simulink model "IntegratedStarterGenerator"  (R2024b)
settings: Solver=ode23tb  StartTime=0.0  StopTime=10  FixedStep=1e-6  RelTol=1e-4  EnableMultiTasking=on
PreLoadFcn:
  | BeltStarterGeneratorData;
model workspace (MAT data in the model file):
  Cdc = 0.001
  ID_MAP = [-155.095933536 -155.095933536 -155.095933536 -155.095933536 -155.095933536 -155.095933536 -155.095933536 -155.095933536 -200.847752045 -245.560073478 -288.511134519 -330.698372533 ... (48076 elements, 28x101x17)]
  IQ_MAP = [-234.678365656 -234.678365656 -234.678365656 -234.678365656 -234.678365656 -234.678365656 -234.678365656 -234.678365656 -207.892729616 -187.030522468 -170.586354015 -157.025794022 ... (48076 elements, 28x101x17)]
  Ki_dcdc = 10
  Ki_id = 170
  Ki_iq = 170
  Ki_vdc = 100
  Kp_dcdc = 0.5
  Kp_id = 0.24
  Kp_iq = 0.24
  Kp_vdc = 20
  L0 = 5e-05
  Ld = 0.00011
  Lq = 0.00011
  Pmax = 140
  RPM_VECT = [0 1000 2000 3000 4000 5000 6000 7000 8000 9000 10000]
  R_f = Simulink.Parameter
  R_f.Value = 1
  R_f.Complexity = 'real'
  R_f.Dimensions = [1 1]
  R_f.DataType = 'auto'
  Rs = 0.085
  TQ_VECT = [-3.5 -3.43 -3.36 -3.29 -3.22 -3.15 -3.08 -3.01 -2.94 -2.87 -2.8 -2.73 -2.66 -2.59 -2.52 -2.45 -2.38 -2.31 -2.24 -2.17 -2.1 -2.03 -1.96 -1.89 -1.82 -1.75 -1.68 -1.61 -1.54 -1.47 -1.4 -1.33 -1.26 -1.19 -1.12 -1.05 -0.98 -0.91 -0.84 -0.77 -0.7 -0.63 -0.56 -0.49 -0.42 -0.35 -0.28 -0.21 -0.14 -0.07 0 0.07 0.14 0.21 0.28 0.35 0.42 0.49 0.56 0.63 0.7 0.77 0.84 0.91 0.98 1.05 1.12 1.19 1.26 1.33 1.4 1.47 1.54 1.61 1.68 1.75 1.82 1.89 1.96 2.03 2.1 2.17 2.24 2.31 2.38 2.45 2.52 2.59 2.66 2.73 2.8 2.87 2.94 3.01 3.08 3.15 3.22 3.29 3.36 3.43 3.5]
  Tmax = 3.5
  Ts = 5e-06
  Tsi = 0.0001
  VDC_VECT = [8 8.625 9.25 9.875 10.5 11.125 11.75 12.375 13 13.625 14.25 14.875 15.5 16.125 16.75 17.375 18]
  dend_id = [1 -0.966796355036]
  dend_iq = [1 -0.900395111642]
  fsw = 5000
  fswd = 5000
  numd_id = 0.0332036449638
  numd_iq = 0.099604888358
  p = 3
  psim = 0.0159
  r_tire = Simulink.Parameter
  r_tire.Value = 0.28
  r_tire.Complexity = 'real'
  r_tire.Dimensions = [1 1]
  r_tire.DataType = 'auto'
  r_tire.DocUnits = 'm'
  tout = [0 5e-06 1e-05 1.5e-05 2e-05 2.5e-05 3e-05 3.5e-05 4e-05 4.5e-05 5e-05 5.5e-05 ... (200005 elements, 200005x1)]
undefined symbols (not defined in the file or in its folder): DiscIntNeverNeededParam
libraries: fl_lib x51, nesl_utility x25, simulink x7, ee_lib x5, eeDiscretePi x3, eeTransforms x2, sdl_lib x1, batteryecm_lib x1, eePmsmCurrentController x1, eePmsmCurrentReferenceGen x1, eePmsmTorqueEstimator x1, eePwmGeneratorTwoLevel x1
(part 1 of 3)
CloseFcn:
  | try,close(h1_BeltStarterGenerator),end
  | clear h1_BeltStarterGenerator
  | 
  | clear simlog_BeltStarterGenerator
  | clear logsout_BeltStarterGenerator
Description:
  | Energy Balance in a 48V Starter Generator
settings Model: SimulationMode=accelerator  Creator=The MathWorks, Inc.  LastModifiedBy=Ujjal.Ghosh
settings SolverCC: MaxConsecutiveZCs=100  AlgebraicLoopSolver=TrustRegion  AutoInsertRateTranBlk=on  MinimalZcImpactIntegration=on  EnableFixedStepZeroCrossing=on  MaxZcPerStep=1
settings DataIOCC: MaxDataPoints=110000  ReturnWorkspaceOutputs=off  SignalLoggingName=logsout_BeltStarterGenerator
settings OptimizationCC: ReuseModelBlockBuffer=off  LifeSpan=inf
settings DebuggingCC: UnderspecifiedInitializationDetection=Classic  MergeDetectMultiDrivingBlocksExec=none  MaxConsecutiveZCsMsg=warning  IgnoredZcDiagnostic=none  UnconnectedInputMsg=warning  UnconnectedOutputMsg=warning  UnconnectedLineMsg=warning  SFUnexpectedBacktrackingDiag=warning  SFNoUnconditionalDefaultTransitionDiag=warning  SFExecutionAtInitializationDiag=none  ArithmeticOperatorsInVariantConditions=warning
settings ModelReferenceCC: EnableRefExpFcnMdlSchedulingChecks=on
settings SFSimCC: SimUseLocalCustomCode=off  CustomCodeUndefinedFunction=UseInterfaceOnly
settings RTWCC: RTWUseLocalCustomCode=off  GPUComputeCapability=3.5  DLArmComputeVersion=19.05
settings CodeAppCC: StateflowObjectComments=on
settings GRTTargetCC: TargetLangStandard=C89/C90 (ANSI)
settings ConfigComp: CovMetricSettings=dw  CovSaveCumulativeToWorkspaceVar=on  CovSaveSingleToWorkspaceVar=on  CovExternalEMLEnable=off
settings SimscapeCC: SimscapeLogSimulationStatistics=on  SimscapeLogToSDI=on  SimscapeLogName=simlog_IntegratedStarterGenerator  SimscapeLogDataHistory=110000

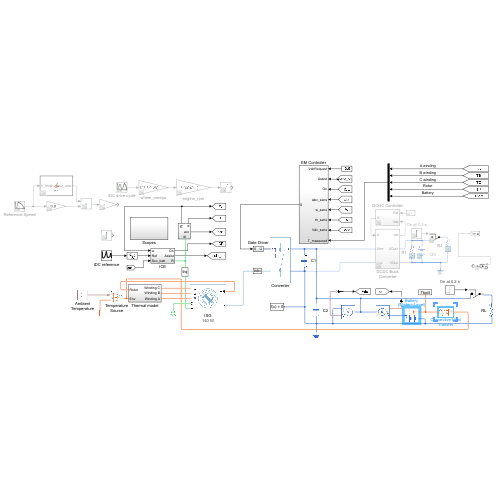
[thumbnail: Simulink's stored preview of the top-level diagram]
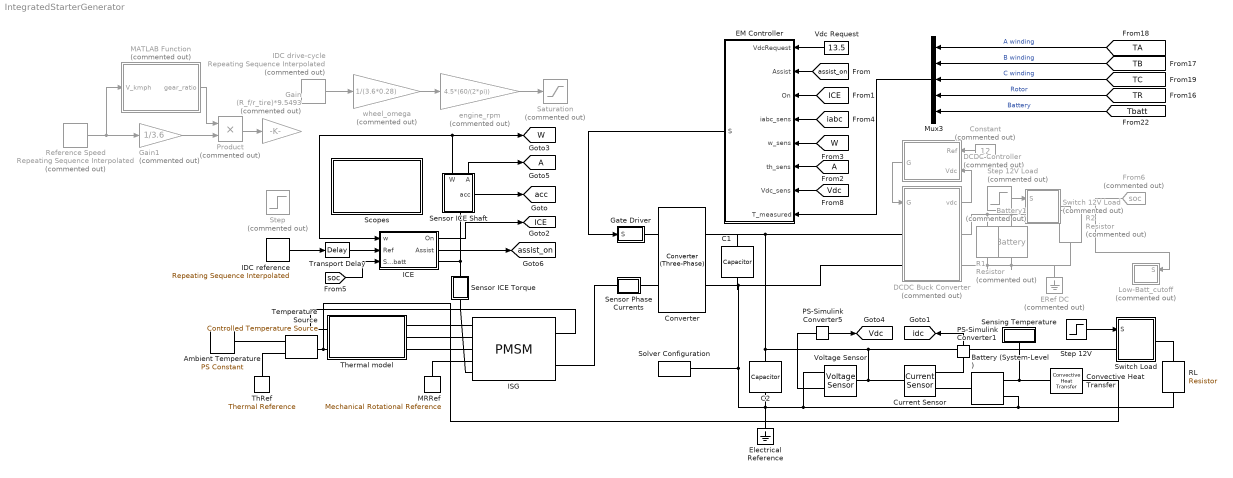
== system IntegratedStarterGenerator ==
  Ambient Temperature : fl_lib/Physical Signals/Sources/PS Constant  constant=312 K
  Battery (System-Level) : sdl_lib/Sources/Battery (System-Level)  Vnom=12 V  R1=45 mOhm  prm_AH=sdl.enum.InfiniteFinite.Finite  AH=3 A*hr  V1=11.8 V  AH1=0.3 A*hr  prm_R2=sdl.enum.DisabledEnabled.Disabled  R2=2000 Ohm  thermal_port=simscape.enum.thermaleffects.model  thermal_mass=4.2 J/K  i_specify=off  i_priority=None  i=0 A  i_nominal_specify=off  i_nominal_value=1  i_nominal_unit=A  v_specify=off  v_priority=None  v=0 V  v_nominal_specify=off  v_nominal_value=1  v_nominal_unit=V  charge_specify=off  charge_priority=High  charge=50 A*hr  charge_nominal_specify=off  charge_nominal_value=1  charge_nominal_unit=A*hr  temperature_specify=on  temperature_priority=Low  temperature=30 degC  temperature_nominal_specify=off  temperature_nominal_value=1  temperature_nominal_unit=K
      settings: InternalSimscapePortConfiguration="{\"Bottom\":[],\"Left\":[{\"id\":\"p\",\"label\":\"+\",\"type\":\"foundation.electrical.electrical\"}],\"Right\":[{\"id\":\"n\",\"label\":\"-\",\"type\":\"foundation.electrical.electrical\"},{\"id\":\"H\",\"label\":\"H\",\"type\":\"foundation.thermal.thermal\"}],\"Top\":[]}"
  Battery1 : batteryecm_lib/Battery  Commented=on  Vnom=12 V  prm_dir=1  R1_dis=2 Ohm  R1_ch=2 Ohm  R1=0.1 Ohm  prm_AH=1  AH=50 hr*A  V1=11.5 V  AH1=25 hr*A  prm_R2=1  R2=inf Ohm  Tmeas=298.15 K  charge_measurement_port=simscape.enum.battery.enable.no  prm_dyn=1  Rp1=0.005 Ohm  tau1=30 s  Rp2=0.005 Ohm  tau2=30 s  Rp3=0.005 Ohm  tau3=30 s  Rp4=0.005 Ohm  tau4=30 s  Rp5=0.005 Ohm  tau5=30 s  prm_fade=1  N_fade=100  AH_fade=45 hr*A  R1_fade=2.02 Ohm  R1_ch_fade=2.02 Ohm  V1_fade=10.35 V  prm_age=1  prm_age_OCV=1  OCV_age=0.9  SOC_age=60  Tmeas_age=298.15 K  delta_time_age_vec=[0] d  temperature_age_vec=[273] K  OCV_scaling_age=2.2134e6  OCV_offset_age=1.632e6  temp_exp_age=0.515833569 V  t_exp_age=0.75  Vnom_T2=12 V  R1_T2=2.2 Ohm  R1_T2_dis=2.2 Ohm  R1_T2_ch=2.2 Ohm  V1_T2=11.4 V  R2_T2=2200 Ohm  Rp1_T2=0.005 Ohm  tau1_T2=30 s  Rp2_T2=0.005 Ohm  tau2_T2=30 s  Rp3_T2=0.005 Ohm  tau3_T2=30 s  Rp4_T2=0.005 Ohm  tau4_T2=30 s  Rp5_T2=0.005 Ohm  tau5_T2=30 s  Tmeas2=273.15 K  thermal_port=simscape.enum.thermaleffects.omit  thermal_mass=30000 J/K  i_specify=off  i_priority=None  i=0 A  i_nominal_specify=off  i_nominal_value=1  i_nominal_unit=A  v_specify=off  v_priority=None  v=0 V  v_nominal_specify=off  v_nominal_value=1  v_nominal_unit=V  charge_specify=on  charge_priority=High  charge=40 hr*A  charge_nominal_specify=off  charge_nominal_value=1  charge_nominal_unit=A*hr  num_cycles_specify=off  num_cycles_priority=High  num_cycles=0  num_cycles_nominal_specify=off  num_cycles_nominal_value=1  num_cycles_nominal_unit=1  temperature_specify=off  temperature_priority=High  temperature=298.15 K  temperature_nominal_specify=off  temperature_nominal_value=1  temperature_nominal_unit=K
      settings: AttributesFormatString=%<Vnom>%<v_unit>
  C1 : fl_lib/Electrical/Electrical Elements/Capacitor  c=Cdc F  r=1e-6 Ohm  g=0 1/Ohm  i_specify=off  i_priority=None  i=0 A  i_nominal_specify=off  i_nominal_value=1  i_nominal_unit=A  v_specify=on  v_priority=Low  v=12 V  v_nominal_specify=off  v_nominal_value=1  v_nominal_unit=V  vc_specify=on  vc_priority=Low  vc=13.5 V  vc_nominal_specify=off  vc_nominal_value=1  vc_nominal_unit=V
  C2 : fl_lib/Electrical/Electrical Elements/Capacitor  c=Cdc F  r=1e-6 Ohm  g=0 1/Ohm  i_specify=off  i_priority=None  i=0 A  i_nominal_specify=off  i_nominal_value=1  i_nominal_unit=A  v_specify=on  v_priority=Low  v=12 V  v_nominal_specify=off  v_nominal_value=1  v_nominal_unit=V  vc_specify=on  vc_priority=Low  vc=13.5 V  vc_nominal_specify=off  vc_nominal_value=1  vc_nominal_unit=V
  Constant : Constant  Commented=on  Value=12  SampleTime=1e-3
  Convective Heat Transfer : fl_lib/Thermal/Thermal Elements/Convective Heat Transfer  thermal_type=foundation.enum.constant_variable.constant  area=0.02 m^2  heat_tr_coeff=0.2 W/(m^2*K)  min_heat_tr_coeff=20 W/(K*m^2)  T_specify=off  T_priority=None  T=0 K  T_nominal_specify=off  T_nominal_value=1  T_nominal_unit=K  Q_specify=off  Q_priority=None  Q=0 W  Q_nominal_specify=off  Q_nominal_value=1  Q_nominal_unit=W
  Converter : ee_lib/Semiconductors & Converters/Converters/Converter (Three-Phase)  port_option=ee.enum.threePhasePort.composite  fidelity_option=ee.enum.converters.fidelity.detailed  device_type=2  showThermalPort=false  K=0  Vth=0.5 V  Vgt=1 V  Vgt_off=-1 V  Ih=1 A  Vf=0.8 V  Ron=0.001 Ohm  Rds=0.001 Ohm  Goff=1e-5 1/Ohm  Eon_scalar=22.86e-3 J  Eoff_scalar=17.14e-3 J  Eoff_natural_commutation=10e-3 J  Voff=300 V  Iout_scalar=600 A  onCurrentMeasDelay=0 s  useCurrentFromPreviousCycle=false  useVoltageFromPreviousCycle=false  diode_param=2  diode_Vf=0.8 V  diode_Ron=0.001 Ohm  diode_Goff=1e-5 1/Ohm  diode_C=50 nF  diode_iRM=-235 A  diode_iF=300 A  diode_idot=-50 A/us  diode_trr_param=1  diode_trr_factor=3  diode_trr=15 us  diode_Qrr=1.5e+3 s*uA  diode_rec_loss_model=ee.enum.diode.reverseRecoveryModel.fixed  diode_ErecVal=0 J  diode_scaleWithIandV=false  diode_ErecMat=zeros(2, 3) J  diode_TjrecVec=[298.15, 398.15] K  diode_IfrecVec=[.1, 1, 10] A  diode_IrecVal=10 A  diode_VrecVal=10 V  diode_tFilter=1 / 1000 / 100 s  thermal_network_parameterization=ee.enum.thermalNetworkTopology.external  Rth=[.08, .5] K/W  Rth_Cauer=[.08, .1, .5] K/W  Rth_Foster=[.08, .14, .22, .16] K/W  thermal_mass_parameterization=ee.enum.thermalNetwork.timeconstant  thermal_mass=[.01, .5] J/K  thermal_mass_Cauer=[.01, .1, .5] J/K  thermal_mass_Foster=[.001, .005, .05, .5] J/K  thermal_time_constant=[.001, .2] s  thermal_time_constant_Cauer=[.001, .1, .2] s  thermal_time_constant_Foster=[7e-05, .0007, .01, .08] s  thermal_mass_initial_temperatures=[25, 25] degC  thermal_mass_initial_temperatures_Cauer=[25, 25, 25] degC  junction_thermal_mass=0.01 J/K  Tvec_initial_Foster=[25, 25, 25, 25] degC  snubber_type=ee.enum.converters.snubber.exclude  Cs=1e-6 F  Rs=0.1 Ohm  Vce_loss=[0, 150, 300] V
  Current Sensor : fl_lib/Electrical/Electrical Sensors/Current Sensor
  DCDC Buck Converter : Subsystem  Tag=PublishSubsystem  Commented=on
  DCDC Controller : Subsystem  Commented=on
  EM Controller : Subsystem
  ERef DC : fl_lib/Electrical/Electrical Elements/Electrical Reference  Commented=on
  Electrical Reference : fl_lib/Electrical/Electrical Elements/Electrical Reference
  From2 : From  TagVisibility=global
  From6 : From  Commented=on  GotoTag=soc  TagVisibility=global
  Gain : Gain  Commented=on  Gain=(R_f/r_tire)*9.5493
  Gain1 : Gain  Commented=on  Gain=1/3.6
  Gate Driver : Subsystem
  Goto5 : Goto  TagVisibility=global
  ICE : Subsystem
  IDC drive-cycle : simulink/Sources/Repeating Sequence Interpolated  Commented=on  OutValues=[0 20 40 60 40 20 0 30 50 70 50 30 0]';  TimeValues=[0 0.5 1 1.5 2 2.5 3 3.5 4 4.5 5 5.5 6]';  LookUpMeth=Interpolation-Use End Values  tsamp=0.0001  OutMin=[]  OutMax=[]  OutDataTypeStr=double  OutputDataTypeScalingMode=double  OutDataType=fixdt(0,8)  OutScaling=2^-10
  IDC reference : simulink/Sources/Repeating Sequence Interpolated  OutValues=[900 900 1000 1500 2425 1000 1136 2000 1500 900].'  TimeValues=[0 0.35 0.4 0.6 0.8 0.95 1.4 1.6 1.65 1.75].'  LookUpMeth=Interpolation-Use End Values  tsamp=0.0001  OutMin=[]  OutMax=[]  OutDataTypeStr=double  OutputDataTypeScalingMode=double  OutDataType=fixdt(0,8)  OutScaling=2^-10
  ISG : ee_lib/Electromechanical/Permanent Magnet/PMSM  port_option=ee.enum.threePhasePort.composite  winding_type=ee.enum.electromech.statorconfiguration.delta  machine_param=ee.enum.pmsm.parameterization.constant  nPolePairs=p  pmflux_param=1  pm_flux_linkage=psim Wb  torque_constant=0.18 N*m/A  back_emf_constant=0.18 V/(rad/s)  stator_param=1  Ld=Ld H  Lq=Lq H  idVec=[-200, 0, 200] A  iqVec=[-200, 0, 200] A  LdMatrix=0.0002 * ones(3, 3) H  LqMatrix=0.0002 * ones(3, 3) H  PmMatrix=0.1 * ones(3, 3) Wb  ktMatrix=0.18 * ones(3, 3) N*m/A  keMatrix=0.18 * ones(3, 3) V/(rad/s)  L0=L0 H  Ls=0.0002 H  Lm=0.00002 H  Ms=0.00002 H  Rs=Rs Ohm  zero_sequence=ee.enum.park.zerosequence.exclude  axes_param=ee.enum.rotorangle.qaxis  loss_param=ee.enum.ironloss.none  losses_oc=[0, 0, 0] W  losses_sc=[0, 0, 0] W  f_losses=60 Hz  Isc_losses=95 A  J=0 kg*m^2  lam=0 N*m/(rad/s)  i_d_specify=off  i_d_priority=None  i_d=0 A  i_d_nominal_specify=off  i_d_nominal_value=1  i_d_nominal_unit=A  i_q_specify=off  i_q_priority=None  i_q=0 A  i_q_nominal_specify=off  i_q_nominal_value=1  i_q_nominal_unit=A  torque_specify=off  torque_priority=None  torque=0 N*m  torque_nominal_specify=off  torque_nominal_value=1  torque_nominal_unit=N*m  angular_velocity_specify=on  angular_velocity_priority=None  angular_velocity=0 rpm  angular_velocity_nominal_specify=off  angular_velocity_nominal_value=1  angular_velocity_nominal_unit=rpm  angular_position_specify=on  angular_position_priority=Low  angular_position=0 rad  angular_position_nominal_specify=off  angular_position_nominal_value=1  angular_position_nominal_unit=deg  alpha=3.93e-3 1/K  alpha_flux=-0.001 1/K  Tmeas=298.15 K  stator_thermal_mass=1 J/K  rotor_thermal_mass=0.5 J/K  Rm_percent_rotor=90  Rd_percent_rotor=30  temperatureA_specify=off  temperatureA_priority=Low  temperatureA=32 degC  temperatureA_nominal_specify=off  temperatureA_nominal_value=1  temperatureA_nominal_unit=degC  temperatureB_specify=off  temperatureB_priority=Low  temperatureB=32 degC  temperatureB_nominal_specify=off  temperatureB_nominal_value=1  temperatureB_nominal_unit=degC  temperatureC_specify=off  temperatureC_priority=Low  temperatureC=32 degC  temperatureC_nominal_specify=off  temperatureC_nominal_value=1  temperatureC_nominal_unit=degC  temperatureR_specify=off  temperatureR_priority=Low  temperatureR=32 degC  temperatureR_nominal_specify=off  temperatureR_nominal_value=1  temperatureR_nominal_unit=degC
      settings: AttributesFormatString=140 W  InternalSimscapePortConfiguration="{\"Bottom\":[],\"Left\":[{\"id\":\"N\",\"label\":\"~\",\"type\":\"foundation.electrical.three_phase\"},{\"id\":\"HR\",\"label\":\"HR\",\"type\":\"foundation.thermal.thermal\"}],\"Right\":[{\"id\":\"R\",\"label\":\"R\",\"type\":\"foundation.mechanical.rotational.rotational\"},{\"id\":\"C\",\"label\":\"C\",\"type\":\"foundation.mechanical.rotational.rotational\"},{\"id\":\"HA\",\"label\":\"HA\",\"type\":\"foundation.thermal.thermal\"},{\"id\":\"HB\",\"label\":\"HB\",\"type\":\"foundation.thermal.thermal\"},{\"id\":\"HC\",\"label\":\"HC\",\"type\":\"foundation.thermal.thermal\"}],\"Top\":[]}"
  Low-Batt_cutoff : Subsystem  Commented=on
      mask Display:
      | patch(-[178.308949107304;178.270428219378;178.155236532808;177.964483406507;177.700005897356;177.364351068347;176.960751458971;176.493093954097;175.965882351142;175.384193986049;174.753630835755;174.080265568098;173.370583058705;172.631417938094;171.869888770445;171.093329497935;170.309218810871;169.525108123807;168.748548851298;167.987019683648;167.247854563037;166.538172053645;165.864806785988;165.234243635694;164.6525552706;164.125343667646;163.657686162771;163.254086553395;162.918431724386;162.653954215236;162.463201088934;162.348009402364;162.309488514438;162.348009402364;162.463201088934;162.653954215236;162.918431724386;163.254086553395;163.657686162771;164.125343667646;164.6525552706;165.234243635694;165.864806785988;166.538172053645;167.247854563037;167.987019683648;168.748548851298;169.525108123807;170.309218810871;171.093329497935;171.869888770445;172.631417938094;173.370583058705;174.080265568098;174.753630835754;175.384193986049;175.965882351142;176.493093954096;176.960751458971;177.364351068347;177.700005897356;177.964483406507;178.155236532808;178.270428219378;178.308949107304;178.308949107304], [113.618216710165;112.834106023101;112.057546750592;111.296017582942;110.556852462331;109.847169952939;109.173804685282;108.543241534988;107.961553169894;107.43434156694;106.966684062065;106.563084452689;106.22742962368;105.962952114529;105.772198988228;105.657007301658;105.618486413732;105.657007301658;105.772198988228;105.962952114529;106.22742962368;106.563084452689;106.966684062065;107.43434156694;107.961553169894;108.543241534988;109.173804685282;109.847169952939;110.556852462331;111.296017582942;112.057546750592;112.834106023101;113.618216710165;114.402327397229;115.178886669738;115.940415837388;116.679580957999;117.389263467392;118.062628735048;118.693191885343;119.274880250436;119.80209185339;120.269749358265;120.673348967641;121.00900379665;121.273481305801;121.464234432102;121.579426118672;121.617947006598;121.579426118672;121.464234432102;121.273481305801;121.00900379665;120.673348967641;120.269749358265;119.80209185339;119.274880250436;118.693191885343;118.062628735048;117.389263467392;116.679580957999;115.940415837388;115.178886669738;114.402327397229;113.618216710165;113.618216710165], [0;0;0])
      | plot(-[178.308949107304;178.270428219378;178.155236532808;177.964483406507;177.700005897356;177.364351068347;176.960751458971;176.493093954097;175.965882351142;175.384193986049;174.753630835755;174.080265568098;173.370583058705;172.631417938094;171.869888770445;171.093329497935;170.309218810871;169.525108123807;168.748548851298;167.987019683648;167.247854563037;166.538172053645;165.864806785988;165.234243635694;164.6525552706;164.125343667646;163.657686162771;163.254086553395;162.918431724386;162.653954215236;162.463201088934;162.348009402364;162.309488514438;162.348009402364;162.463201088934;162.653954215236;162.918431724386;163.254086553395;163.657686162771;164.125343667646;164.6525552706;165.234243635694;165.864806785988;166.538172053645;167.247854563037;167.987019683648;168.748548851298;169.525108123807;170.309218810871;171.093329497935;171.869888770445;172.631417938094;173.370583058705;174.080265568098;174.753630835754;175.384193986049;175.965882351142;176.493093954096;176.960751458971;177.364351068347;177.700005897356;177.964483406507;178.155236532808;178.270428219378;178.308949107304;178.308949107304], [113.618216710165;112.834106023101;112.057546750592;111.296017582942;110.556852462331;109.847169952939;109.173804685282;108.543241534988;107.961553169894;107.43434156694;106.966684062065;106.563084452689;106.22742962368;105.962952114529;105.772198988228;105.657007301658;105.618486413732;105.657007301658;105.772198988228;105.962952114529;106.22742962368;106.563084452689;106.966684062065;107.43434156694;107.961553169894;108.543241534988;109.173804685282;109.847169952939;110.556852462331;111.296017582942;112.057546750592;112.834106023101;113.618216710165;114.402327397229;115.178886669738;115.940415837388;116.679580957999;117.389263467392;118.062628735048;118.693191885343;119.274880250436;119.80209185339;120.269749358265;120.673348967641;121.00900379665;121.273481305801;121.464234432102;121.579426118672;121.617947006598;121.579426118672;121.464234432102;121.273481305801;121.00900379665;120.673348967641;120.269749358265;119.80209185339;119.274880250436;118.693191885343;118.062628735048;117.389263467392;116.679580957999;115.940415837388;115.178886669738;114.402327397229;113.618216710165;113.618216710165])
      | patch(-[64.926944905892;64.888424017966;64.7732323313963;64.5824792050947;64.3180016959439;63.9823468669351;63.5787472575591;63.1110897526843;62.5838781497303;62.0021897846366;61.3716266343423;60.6982613666856;59.988578857293;59.2494137366818;58.4878845690323;57.7113252965232;56.927214609459;56.1431039223949;55.3665446498857;54.6050154822362;53.8658503616251;53.1561678522324;52.4828025845758;51.8522394342815;51.2705510691878;50.7433394662337;50.275681961359;49.872082351983;49.5364275229742;49.2719500138234;49.0811968875218;48.9660052009521;48.9274843130261;48.9660052009521;49.0811968875218;49.2719500138234;49.5364275229742;49.8720823519831;50.275681961359;50.7433394662338;51.2705510691878;51.8522394342816;52.4828025845758;53.1561678522325;53.8658503616251;54.6050154822362;55.3665446498858;56.143103922395;56.927214609459;57.7113252965232;58.4878845690323;59.2494137366818;59.988578857293;60.6982613666856;61.3716266343422;62.0021897846366;62.5838781497303;63.1110897526843;63.5787472575591;63.982346866935;64.3180016959439;64.5824792050947;64.7732323313963;64.888424017966;64.926944905892;64.926944905892], [113.618216710165;112.834106023101;112.057546750592;111.296017582942;110.556852462331;109.847169952939;109.173804685282;108.543241534988;107.961553169894;107.43434156694;106.966684062065;106.563084452689;106.22742962368;105.962952114529;105.772198988228;105.657007301658;105.618486413732;105.657007301658;105.772198988228;105.962952114529;106.22742962368;106.563084452689;106.966684062065;107.43434156694;107.961553169894;108.543241534988;109.173804685282;109.847169952939;110.556852462331;111.296017582942;112.057546750592;112.834106023101;113.618216710165;114.402327397229;115.178886669738;115.940415837388;116.679580957999;117.389263467392;118.062628735048;118.693191885343;119.274880250436;119.80209185339;120.269749358265;120.673348967641;121.00900379665;121.273481305801;121.464234432102;121.579426118672;121.617947006598;121.579426118672;121.464234432102;121.273481305801;121.00900379665;120.673348967641;120.269749358265;119.80209185339;119.274880250436;118.693191885343;118.062628735048;117.389263467392;116.679580957999;115.940415837388;115.178886669738;114.402327397229;113.618216710165;113.618216710165], [0;0;0])
      | plot(-[64.926944905892;64.888424017966;64.7732323313963;64.5824792050947;64.3180016959439;63.9823468669351;63.5787472575591;63.1110897526843;62.5838781497303;62.0021897846366;61.3716266343423;60.6982613666856;59.988578857293;59.2494137366818;58.4878845690323;57.7113252965232;56.927214609459;56.1431039223949;55.3665446498857;54.6050154822362;53.8658503616251;53.1561678522324;52.4828025845758;51.8522394342815;51.2705510691878;50.7433394662337;50.275681961359;49.872082351983;49.5364275229742;49.2719500138234;49.0811968875218;48.9660052009521;48.9274843130261;48.9660052009521;49.0811968875218;49.2719500138234;49.5364275229742;49.8720823519831;50.275681961359;50.7433394662338;51.2705510691878;51.8522394342816;52.4828025845758;53.1561678522325;53.8658503616251;54.6050154822362;55.3665446498858;56.143103922395;56.927214609459;57.7113252965232;58.4878845690323;59.2494137366818;59.988578857293;60.6982613666856;61.3716266343422;62.0021897846366;62.5838781497303;63.1110897526843;63.5787472575591;63.982346866935;64.3180016959439;64.5824792050947;64.7732323313963;64.888424017966;64.926944905892;64.926944905892], [113.618216710165;112.834106023101;112.057546750592;111.296017582942;110.556852462331;109.847169952939;109.173804685282;108.543241534988;107.961553169894;107.43434156694;106.966684062065;106.563084452689;106.22742962368;105.962952114529;105.772198988228;105.657007301658;105.618486413732;105.657007301658;105.772198988228;105.962952114529;106.22742962368;106.563084452689;106.966684062065;107.43434156694;107.961553169894;108.543241534988;109.173804685282;109.847169952939;110.556852462331;111.296017582942;112.057546750592;112.834106023101;113.618216710165;114.402327397229;115.178886669738;115.940415837388;116.679580957999;117.389263467392;118.062628735048;118.693191885343;119.274880250436;119.80209185339;120.269749358265;120.673348967641;121.00900379665;121.273481305801;121.464234432102;121.579426118672;121.617947006598;121.579426118672;121.464234432102;121.273481305801;121.00900379665;120.673348967641;120.269749358265;119.80209185339;119.274880250436;118.693191885343;118.062628735048;117.389263467392;116.679580957999;115.940415837388;115.178886669738;114.402327397229;113.618216710165;113.618216710165])
      | plot(-[56.927214609459;161.805568495765], [113.618216710165;56.927214609459])
      | plot(-[227.000220911577;113.618216710165;113.618216710165], [170.309218810871;170.309218810871;82.4381655547768])
      | patch(-[0;227.23643342033;227.23643342033;0;0;0.472425017505884;0.472425017505884;226.764008402824;226.764008402824;0.472425017505884;0], [227.23643342033;227.23643342033;0;0;227.23643342033;226.764008402824;0.472425017505884;0.472425017505884;226.764008402824;226.764008402824;227.23643342033], [1;1;1])
      | plot(-[170.309218810871;198.654719861224;198.654719861224;227.000220911577], [113.618216710165;113.618216710165;56.927214609459;56.927214609459])
      | plot(-[56.927214609459;0.236212508752942], [113.618216710165;113.618216710165])
  MATLAB Function : MATLAB Function  Commented=on  TreatAsAtomicUnit=on
  MRRef : fl_lib/Mechanical/Rotational Elements/Mechanical Rotational Reference
  Mux3 : Mux  Inputs=5
  PS-Simulink Converter1 : nesl_utility/PS-Simulink Converter  PhysicalDomain=network_engine_domain  SubClassName=ps_output  LeftPortType=input  RightPortType=output  PseudoPeriodic=off  Frequencies=[]  VectorFormat=1-D array  Unit=A  AffineConversion=off
  PS-Simulink Converter5 : nesl_utility/PS-Simulink Converter  PhysicalDomain=network_engine_domain  SubClassName=ps_output  LeftPortType=input  RightPortType=output  PseudoPeriodic=off  Frequencies=[]  VectorFormat=1-D array  Unit=V  AffineConversion=off
  Product : Product  Commented=on
  R1 : fl_lib/Electrical/Electrical Elements/Resistor  Commented=on  R=1 Ohm  i_specify=off  i_priority=None  i=0 A  i_nominal_specify=off  i_nominal_value=1  i_nominal_unit=A  v_specify=off  v_priority=None  v=0 V  v_nominal_specify=off  v_nominal_value=1  v_nominal_unit=V
  R2 : fl_lib/Electrical/Electrical Elements/Resistor  Commented=on  R=1 Ohm  i_specify=off  i_priority=None  i=0 A  i_nominal_specify=off  i_nominal_value=1  i_nominal_unit=A  v_specify=off  v_priority=None  v=0 V  v_nominal_specify=off  v_nominal_value=1  v_nominal_unit=V
  RL : fl_lib/Electrical/Electrical Elements/Resistor  R=10 Ohm  i_specify=off  i_priority=None  i=0 A  i_nominal_specify=off  i_nominal_value=1  i_nominal_unit=A  v_specify=off  v_priority=None  v=0 V  v_nominal_specify=off  v_nominal_value=1  v_nominal_unit=V
  Reference Speed : simulink/Sources/Repeating Sequence Interpolated  Commented=on  OutValues=[0 0 10 20 30 20 10 0].'  TimeValues=[0 0.1 0.2 0.25 0.3 0.65 0.85 1].'  LookUpMeth=Interpolation-Use End Values  tsamp=0.0001  OutMin=[]  OutMax=[]  OutDataTypeStr=double  OutputDataTypeScalingMode=double  OutDataType=fixdt(0,8)  OutScaling=2^-10
  Saturation : Saturate  Commented=on  UpperLimit=2500  LowerLimit=900  LinearizeAsGain=off  ZeroCross=off
  Scopes : Subsystem
  Sensing Temperature : Subsystem
      mask Display: disp('Tbatt')
  Sensor ICE Torque : Subsystem
      mask Display: disp('trq')
  Sensor ICE Shaft : Subsystem
      settings: PortSchema="{\"entries\":[{\"content\":{\"sides\":[{\"content\":{\"connectorIds\":[\"LConn1\"]},\"type\":\"ConnectorPlacement.EquallySpacedRectSide\",\"uuid\":\"3e5e68ec-a87c-42a5-a11e-b99611e4de8d\"},{\"content\":{\"connectorIds\":[\"Out1\",\"Out2\"],\"side\":\"RIGHT\"},\"type\":\"ConnectorPlacement.EquallySpacedRectSide\",\"uuid\":\"c8d9cc5c-950c-420c-a9c5-7484f9c0881e\"},{\"content\":{\"side\":\"TOP\"},\"type\":\"ConnectorPlacement.EquallySpacedRectSide\",\"uuid\":\"2fd89d58-252b-4c79-93f0-b9e45502d9f0\"},{\"content\":{\"connectorIds\":[\"Out3\"],\"side\":\"BOTTOM\"},\"type\":\"ConnectorPlacement.EquallySpacedRectSide\",\"uuid\":\"fea9b83b-c277-4256-afb9-2e7ef8af4caa\"}]},\"type\":\"ConnectorPlacement.EquallySpacedConnector\",\"uuid\":\"8d4a9bec-8b5e-4fd7-a708-99a7103a3dd0\"}],\"packageUris\":[\"http://schema.mathworks.com/mf0/Connector/R2020b\"],\"version\":\"1.0\"}"
  Sensor Phase Currents : Subsystem
      mask Display: disp('iabc')
  Solver Configuration : nesl_utility/Solver Configuration  PhysicalDomain=network_engine_domain  SubClassName=solver  LeftPortType=input  RightPortType=generic  Tones=[]  Harmonics=[]  SimulateNoise=off  Profile=off  UseLocalSampling=off  EnableSwitchedLinearOptims=on  FrequencyDomain=off  UseCCode=off  RelTol=0.001  AbsTol=1e-06  MinStep=1e-09  ToWorkspace=off  RevertToSquareIcSolve=off  NumHomotopyIterations=100  PhasorMode=off  PhasorModeNumHarmonics=1  ConsistencySolver=NEWTON_FTOL  IndexReductionMethod=DerivativeReplacement  DoDC=off  ResidualTolerance=1e-4  ConsistencyTolSource=GLOBAL  ConsistencyAbsTol=0.001  ConsistencyRelTol=0.001  ConsistencyTolFactor=0.001  UseLocalSolver=on  LocalSolverChoice=NE_BACKWARD_EULER_ADVANCER  ResolveIndetEquations=on  FunctionEvalNumThread=1  LocalSolverSampleTime=Ts  DoFixedCost=on  MaxNonlinIter=3  MaxModeIter=2  ComputeImpulses=off  ImpulseIterations=2  LinearAlgebra=auto  LinearAlgebraNumThread=0  EquationFormulation=NE_TIME_EF  DelaysMemoryBudget=1024  AutomaticFiltering=on  FilteringTimeConstant=0.001  PartitionStorageMethod=AS_NEEDED  PartitionMemoryBudget=1024  PartitionMethod=FAST  MultibodyUseLocalSolver=off  MultibodyLocalSolverChoice=ODE1  MultibodyLocalSolverSampleTime=0.001
  Step : Step  Commented=on  Time=0.05  After=900  SampleTime=0.01
  Step 12V : Step  Time=0.2  SampleTime=0
      settings: AttributesFormatString=On at %<Time> s
  Step 12V Load : Step  Commented=on  Time=0.3  SampleTime=0
      settings: AttributesFormatString=On at %<Time> s
  Switch 12V Load : Subsystem  Commented=on
      mask Display:
      | patch(-[178.308949107304;178.270428219378;178.155236532808;177.964483406507;177.700005897356;177.364351068347;176.960751458971;176.493093954097;175.965882351142;175.384193986049;174.753630835755;174.080265568098;173.370583058705;172.631417938094;171.869888770445;171.093329497935;170.309218810871;169.525108123807;168.748548851298;167.987019683648;167.247854563037;166.538172053645;165.864806785988;165.234243635694;164.6525552706;164.125343667646;163.657686162771;163.254086553395;162.918431724386;162.653954215236;162.463201088934;162.348009402364;162.309488514438;162.348009402364;162.463201088934;162.653954215236;162.918431724386;163.254086553395;163.657686162771;164.125343667646;164.6525552706;165.234243635694;165.864806785988;166.538172053645;167.247854563037;167.987019683648;168.748548851298;169.525108123807;170.309218810871;171.093329497935;171.869888770445;172.631417938094;173.370583058705;174.080265568098;174.753630835754;175.384193986049;175.965882351142;176.493093954096;176.960751458971;177.364351068347;177.700005897356;177.964483406507;178.155236532808;178.270428219378;178.308949107304;178.308949107304], [113.618216710165;112.834106023101;112.057546750592;111.296017582942;110.556852462331;109.847169952939;109.173804685282;108.543241534988;107.961553169894;107.43434156694;106.966684062065;106.563084452689;106.22742962368;105.962952114529;105.772198988228;105.657007301658;105.618486413732;105.657007301658;105.772198988228;105.962952114529;106.22742962368;106.563084452689;106.966684062065;107.43434156694;107.961553169894;108.543241534988;109.173804685282;109.847169952939;110.556852462331;111.296017582942;112.057546750592;112.834106023101;113.618216710165;114.402327397229;115.178886669738;115.940415837388;116.679580957999;117.389263467392;118.062628735048;118.693191885343;119.274880250436;119.80209185339;120.269749358265;120.673348967641;121.00900379665;121.273481305801;121.464234432102;121.579426118672;121.617947006598;121.579426118672;121.464234432102;121.273481305801;121.00900379665;120.673348967641;120.269749358265;119.80209185339;119.274880250436;118.693191885343;118.062628735048;117.389263467392;116.679580957999;115.940415837388;115.178886669738;114.402327397229;113.618216710165;113.618216710165], [0;0;0])
      | plot(-[178.308949107304;178.270428219378;178.155236532808;177.964483406507;177.700005897356;177.364351068347;176.960751458971;176.493093954097;175.965882351142;175.384193986049;174.753630835755;174.080265568098;173.370583058705;172.631417938094;171.869888770445;171.093329497935;170.309218810871;169.525108123807;168.748548851298;167.987019683648;167.247854563037;166.538172053645;165.864806785988;165.234243635694;164.6525552706;164.125343667646;163.657686162771;163.254086553395;162.918431724386;162.653954215236;162.463201088934;162.348009402364;162.309488514438;162.348009402364;162.463201088934;162.653954215236;162.918431724386;163.254086553395;163.657686162771;164.125343667646;164.6525552706;165.234243635694;165.864806785988;166.538172053645;167.247854563037;167.987019683648;168.748548851298;169.525108123807;170.309218810871;171.093329497935;171.869888770445;172.631417938094;173.370583058705;174.080265568098;174.753630835754;175.384193986049;175.965882351142;176.493093954096;176.960751458971;177.364351068347;177.700005897356;177.964483406507;178.155236532808;178.270428219378;178.308949107304;178.308949107304], [113.618216710165;112.834106023101;112.057546750592;111.296017582942;110.556852462331;109.847169952939;109.173804685282;108.543241534988;107.961553169894;107.43434156694;106.966684062065;106.563084452689;106.22742962368;105.962952114529;105.772198988228;105.657007301658;105.618486413732;105.657007301658;105.772198988228;105.962952114529;106.22742962368;106.563084452689;106.966684062065;107.43434156694;107.961553169894;108.543241534988;109.173804685282;109.847169952939;110.556852462331;111.296017582942;112.057546750592;112.834106023101;113.618216710165;114.402327397229;115.178886669738;115.940415837388;116.679580957999;117.389263467392;118.062628735048;118.693191885343;119.274880250436;119.80209185339;120.269749358265;120.673348967641;121.00900379665;121.273481305801;121.464234432102;121.579426118672;121.617947006598;121.579426118672;121.464234432102;121.273481305801;121.00900379665;120.673348967641;120.269749358265;119.80209185339;119.274880250436;118.693191885343;118.062628735048;117.389263467392;116.679580957999;115.940415837388;115.178886669738;114.402327397229;113.618216710165;113.618216710165])
      | patch(-[64.926944905892;64.888424017966;64.7732323313963;64.5824792050947;64.3180016959439;63.9823468669351;63.5787472575591;63.1110897526843;62.5838781497303;62.0021897846366;61.3716266343423;60.6982613666856;59.988578857293;59.2494137366818;58.4878845690323;57.7113252965232;56.927214609459;56.1431039223949;55.3665446498857;54.6050154822362;53.8658503616251;53.1561678522324;52.4828025845758;51.8522394342815;51.2705510691878;50.7433394662337;50.275681961359;49.872082351983;49.5364275229742;49.2719500138234;49.0811968875218;48.9660052009521;48.9274843130261;48.9660052009521;49.0811968875218;49.2719500138234;49.5364275229742;49.8720823519831;50.275681961359;50.7433394662338;51.2705510691878;51.8522394342816;52.4828025845758;53.1561678522325;53.8658503616251;54.6050154822362;55.3665446498858;56.143103922395;56.927214609459;57.7113252965232;58.4878845690323;59.2494137366818;59.988578857293;60.6982613666856;61.3716266343422;62.0021897846366;62.5838781497303;63.1110897526843;63.5787472575591;63.982346866935;64.3180016959439;64.5824792050947;64.7732323313963;64.888424017966;64.926944905892;64.926944905892], [113.618216710165;112.834106023101;112.057546750592;111.296017582942;110.556852462331;109.847169952939;109.173804685282;108.543241534988;107.961553169894;107.43434156694;106.966684062065;106.563084452689;106.22742962368;105.962952114529;105.772198988228;105.657007301658;105.618486413732;105.657007301658;105.772198988228;105.962952114529;106.22742962368;106.563084452689;106.966684062065;107.43434156694;107.961553169894;108.543241534988;109.173804685282;109.847169952939;110.556852462331;111.296017582942;112.057546750592;112.834106023101;113.618216710165;114.402327397229;115.178886669738;115.940415837388;116.679580957999;117.389263467392;118.062628735048;118.693191885343;119.274880250436;119.80209185339;120.269749358265;120.673348967641;121.00900379665;121.273481305801;121.464234432102;121.579426118672;121.617947006598;121.579426118672;121.464234432102;121.273481305801;121.00900379665;120.673348967641;120.269749358265;119.80209185339;119.274880250436;118.693191885343;118.062628735048;117.389263467392;116.679580957999;115.940415837388;115.178886669738;114.402327397229;113.618216710165;113.618216710165], [0;0;0])
      | plot(-[64.926944905892;64.888424017966;64.7732323313963;64.5824792050947;64.3180016959439;63.9823468669351;63.5787472575591;63.1110897526843;62.5838781497303;62.0021897846366;61.3716266343423;60.6982613666856;59.988578857293;59.2494137366818;58.4878845690323;57.7113252965232;56.927214609459;56.1431039223949;55.3665446498857;54.6050154822362;53.8658503616251;53.1561678522324;52.4828025845758;51.8522394342815;51.2705510691878;50.7433394662337;50.275681961359;49.872082351983;49.5364275229742;49.2719500138234;49.0811968875218;48.9660052009521;48.9274843130261;48.9660052009521;49.0811968875218;49.2719500138234;49.5364275229742;49.8720823519831;50.275681961359;50.7433394662338;51.2705510691878;51.8522394342816;52.4828025845758;53.1561678522325;53.8658503616251;54.6050154822362;55.3665446498858;56.143103922395;56.927214609459;57.7113252965232;58.4878845690323;59.2494137366818;59.988578857293;60.6982613666856;61.3716266343422;62.0021897846366;62.5838781497303;63.1110897526843;63.5787472575591;63.982346866935;64.3180016959439;64.5824792050947;64.7732323313963;64.888424017966;64.926944905892;64.926944905892], [113.618216710165;112.834106023101;112.057546750592;111.296017582942;110.556852462331;109.847169952939;109.173804685282;108.543241534988;107.961553169894;107.43434156694;106.966684062065;106.563084452689;106.22742962368;105.962952114529;105.772198988228;105.657007301658;105.618486413732;105.657007301658;105.772198988228;105.962952114529;106.22742962368;106.563084452689;106.966684062065;107.43434156694;107.961553169894;108.543241534988;109.173804685282;109.847169952939;110.556852462331;111.296017582942;112.057546750592;112.834106023101;113.618216710165;114.402327397229;115.178886669738;115.940415837388;116.679580957999;117.389263467392;118.062628735048;118.693191885343;119.274880250436;119.80209185339;120.269749358265;120.673348967641;121.00900379665;121.273481305801;121.464234432102;121.579426118672;121.617947006598;121.579426118672;121.464234432102;121.273481305801;121.00900379665;120.673348967641;120.269749358265;119.80209185339;119.274880250436;118.693191885343;118.062628735048;117.389263467392;116.679580957999;115.940415837388;115.178886669738;114.402327397229;113.618216710165;113.618216710165])
      | plot(-[56.927214609459;161.805568495765], [113.618216710165;56.927214609459])
      | plot(-[227.000220911577;113.618216710165;113.618216710165], [170.309218810871;170.309218810871;82.4381655547768])
      | patch(-[0;227.23643342033;227.23643342033;0;0;0.472425017505884;0.472425017505884;226.764008402824;226.764008402824;0.472425017505884;0], [227.23643342033;227.23643342033;0;0;227.23643342033;226.764008402824;0.472425017505884;0.472425017505884;226.764008402824;226.764008402824;227.23643342033], [1;1;1])
      | plot(-[170.309218810871;198.654719861224;198.654719861224;227.000220911577], [113.618216710165;113.618216710165;56.927214609459;56.927214609459])
      | plot(-[56.927214609459;0.236212508752942], [113.618216710165;113.618216710165])
  Switch Load : Subsystem
      mask Display:
      | patch(-[178.308949107304;178.270428219378;178.155236532808;177.964483406507;177.700005897356;177.364351068347;176.960751458971;176.493093954097;175.965882351142;175.384193986049;174.753630835755;174.080265568098;173.370583058705;172.631417938094;171.869888770445;171.093329497935;170.309218810871;169.525108123807;168.748548851298;167.987019683648;167.247854563037;166.538172053645;165.864806785988;165.234243635694;164.6525552706;164.125343667646;163.657686162771;163.254086553395;162.918431724386;162.653954215236;162.463201088934;162.348009402364;162.309488514438;162.348009402364;162.463201088934;162.653954215236;162.918431724386;163.254086553395;163.657686162771;164.125343667646;164.6525552706;165.234243635694;165.864806785988;166.538172053645;167.247854563037;167.987019683648;168.748548851298;169.525108123807;170.309218810871;171.093329497935;171.869888770445;172.631417938094;173.370583058705;174.080265568098;174.753630835754;175.384193986049;175.965882351142;176.493093954096;176.960751458971;177.364351068347;177.700005897356;177.964483406507;178.155236532808;178.270428219378;178.308949107304;178.308949107304], [113.618216710165;112.834106023101;112.057546750592;111.296017582942;110.556852462331;109.847169952939;109.173804685282;108.543241534988;107.961553169894;107.43434156694;106.966684062065;106.563084452689;106.22742962368;105.962952114529;105.772198988228;105.657007301658;105.618486413732;105.657007301658;105.772198988228;105.962952114529;106.22742962368;106.563084452689;106.966684062065;107.43434156694;107.961553169894;108.543241534988;109.173804685282;109.847169952939;110.556852462331;111.296017582942;112.057546750592;112.834106023101;113.618216710165;114.402327397229;115.178886669738;115.940415837388;116.679580957999;117.389263467392;118.062628735048;118.693191885343;119.274880250436;119.80209185339;120.269749358265;120.673348967641;121.00900379665;121.273481305801;121.464234432102;121.579426118672;121.617947006598;121.579426118672;121.464234432102;121.273481305801;121.00900379665;120.673348967641;120.269749358265;119.80209185339;119.274880250436;118.693191885343;118.062628735048;117.389263467392;116.679580957999;115.940415837388;115.178886669738;114.402327397229;113.618216710165;113.618216710165], [0;0;0])
      | plot(-[178.308949107304;178.270428219378;178.155236532808;177.964483406507;177.700005897356;177.364351068347;176.960751458971;176.493093954097;175.965882351142;175.384193986049;174.753630835755;174.080265568098;173.370583058705;172.631417938094;171.869888770445;171.093329497935;170.309218810871;169.525108123807;168.748548851298;167.987019683648;167.247854563037;166.538172053645;165.864806785988;165.234243635694;164.6525552706;164.125343667646;163.657686162771;163.254086553395;162.918431724386;162.653954215236;162.463201088934;162.348009402364;162.309488514438;162.348009402364;162.463201088934;162.653954215236;162.918431724386;163.254086553395;163.657686162771;164.125343667646;164.6525552706;165.234243635694;165.864806785988;166.538172053645;167.247854563037;167.987019683648;168.748548851298;169.525108123807;170.309218810871;171.093329497935;171.869888770445;172.631417938094;173.370583058705;174.080265568098;174.753630835754;175.384193986049;175.965882351142;176.493093954096;176.960751458971;177.364351068347;177.700005897356;177.964483406507;178.155236532808;178.270428219378;178.308949107304;178.308949107304], [113.618216710165;112.834106023101;112.057546750592;111.296017582942;110.556852462331;109.847169952939;109.173804685282;108.543241534988;107.961553169894;107.43434156694;106.966684062065;106.563084452689;106.22742962368;105.962952114529;105.772198988228;105.657007301658;105.618486413732;105.657007301658;105.772198988228;105.962952114529;106.22742962368;106.563084452689;106.966684062065;107.43434156694;107.961553169894;108.543241534988;109.173804685282;109.847169952939;110.556852462331;111.296017582942;112.057546750592;112.834106023101;113.618216710165;114.402327397229;115.178886669738;115.940415837388;116.679580957999;117.389263467392;118.062628735048;118.693191885343;119.274880250436;119.80209185339;120.269749358265;120.673348967641;121.00900379665;121.273481305801;121.464234432102;121.579426118672;121.617947006598;121.579426118672;121.464234432102;121.273481305801;121.00900379665;120.673348967641;120.269749358265;119.80209185339;119.274880250436;118.693191885343;118.062628735048;117.389263467392;116.679580957999;115.940415837388;115.178886669738;114.402327397229;113.618216710165;113.618216710165])
      | patch(-[64.926944905892;64.888424017966;64.7732323313963;64.5824792050947;64.3180016959439;63.9823468669351;63.5787472575591;63.1110897526843;62.5838781497303;62.0021897846366;61.3716266343423;60.6982613666856;59.988578857293;59.2494137366818;58.4878845690323;57.7113252965232;56.927214609459;56.1431039223949;55.3665446498857;54.6050154822362;53.8658503616251;53.1561678522324;52.4828025845758;51.8522394342815;51.2705510691878;50.7433394662337;50.275681961359;49.872082351983;49.5364275229742;49.2719500138234;49.0811968875218;48.9660052009521;48.9274843130261;48.9660052009521;49.0811968875218;49.2719500138234;49.5364275229742;49.8720823519831;50.275681961359;50.7433394662338;51.2705510691878;51.8522394342816;52.4828025845758;53.1561678522325;53.8658503616251;54.6050154822362;55.3665446498858;56.143103922395;56.927214609459;57.7113252965232;58.4878845690323;59.2494137366818;59.988578857293;60.6982613666856;61.3716266343422;62.0021897846366;62.5838781497303;63.1110897526843;63.5787472575591;63.982346866935;64.3180016959439;64.5824792050947;64.7732323313963;64.888424017966;64.926944905892;64.926944905892], [113.618216710165;112.834106023101;112.057546750592;111.296017582942;110.556852462331;109.847169952939;109.173804685282;108.543241534988;107.961553169894;107.43434156694;106.966684062065;106.563084452689;106.22742962368;105.962952114529;105.772198988228;105.657007301658;105.618486413732;105.657007301658;105.772198988228;105.962952114529;106.22742962368;106.563084452689;106.966684062065;107.43434156694;107.961553169894;108.543241534988;109.173804685282;109.847169952939;110.556852462331;111.296017582942;112.057546750592;112.834106023101;113.618216710165;114.402327397229;115.178886669738;115.940415837388;116.679580957999;117.389263467392;118.062628735048;118.693191885343;119.274880250436;119.80209185339;120.269749358265;120.673348967641;121.00900379665;121.273481305801;121.464234432102;121.579426118672;121.617947006598;121.579426118672;121.464234432102;121.273481305801;121.00900379665;120.673348967641;120.269749358265;119.80209185339;119.274880250436;118.693191885343;118.062628735048;117.389263467392;116.679580957999;115.940415837388;115.178886669738;114.402327397229;113.618216710165;113.618216710165], [0;0;0])
      | plot(-[64.926944905892;64.888424017966;64.7732323313963;64.5824792050947;64.3180016959439;63.9823468669351;63.5787472575591;63.1110897526843;62.5838781497303;62.0021897846366;61.3716266343423;60.6982613666856;59.988578857293;59.2494137366818;58.4878845690323;57.7113252965232;56.927214609459;56.1431039223949;55.3665446498857;54.6050154822362;53.8658503616251;53.1561678522324;52.4828025845758;51.8522394342815;51.2705510691878;50.7433394662337;50.275681961359;49.872082351983;49.5364275229742;49.2719500138234;49.0811968875218;48.9660052009521;48.9274843130261;48.9660052009521;49.0811968875218;49.2719500138234;49.5364275229742;49.8720823519831;50.275681961359;50.7433394662338;51.2705510691878;51.8522394342816;52.4828025845758;53.1561678522325;53.8658503616251;54.6050154822362;55.3665446498858;56.143103922395;56.927214609459;57.7113252965232;58.4878845690323;59.2494137366818;59.988578857293;60.6982613666856;61.3716266343422;62.0021897846366;62.5838781497303;63.1110897526843;63.5787472575591;63.982346866935;64.3180016959439;64.5824792050947;64.7732323313963;64.888424017966;64.926944905892;64.926944905892], [113.618216710165;112.834106023101;112.057546750592;111.296017582942;110.556852462331;109.847169952939;109.173804685282;108.543241534988;107.961553169894;107.43434156694;106.966684062065;106.563084452689;106.22742962368;105.962952114529;105.772198988228;105.657007301658;105.618486413732;105.657007301658;105.772198988228;105.962952114529;106.22742962368;106.563084452689;106.966684062065;107.43434156694;107.961553169894;108.543241534988;109.173804685282;109.847169952939;110.556852462331;111.296017582942;112.057546750592;112.834106023101;113.618216710165;114.402327397229;115.178886669738;115.940415837388;116.679580957999;117.389263467392;118.062628735048;118.693191885343;119.274880250436;119.80209185339;120.269749358265;120.673348967641;121.00900379665;121.273481305801;121.464234432102;121.579426118672;121.617947006598;121.579426118672;121.464234432102;121.273481305801;121.00900379665;120.673348967641;120.269749358265;119.80209185339;119.274880250436;118.693191885343;118.062628735048;117.389263467392;116.679580957999;115.940415837388;115.178886669738;114.402327397229;113.618216710165;113.618216710165])
      | plot(-[56.927214609459;161.805568495765], [113.618216710165;56.927214609459])
      | plot(-[227.000220911577;113.618216710165;113.618216710165], [170.309218810871;170.309218810871;82.4381655547768])
      | patch(-[0;227.23643342033;227.23643342033;0;0;0.472425017505884;0.472425017505884;226.764008402824;226.764008402824;0.472425017505884;0], [227.23643342033;227.23643342033;0;0;227.23643342033;226.764008402824;0.472425017505884;0.472425017505884;226.764008402824;226.764008402824;227.23643342033], [1;1;1])
      | plot(-[170.309218810871;198.654719861224;198.654719861224;227.000220911577], [113.618216710165;113.618216710165;56.927214609459;56.927214609459])
      | plot(-[56.927214609459;0.236212508752942], [113.618216710165;113.618216710165])
  Temperature Source : fl_lib/Thermal/Thermal Sources/Controlled Temperature Source
  ThRef : fl_lib/Thermal/Thermal Elements/Thermal Reference
  Thermal model : Subsystem  Tag=PublishSubsystem
  Transport Delay : TransportDelay  DelayTime=0.05
  Vdc Request : Constant  Value=13.5
  Voltage Sensor : fl_lib/Electrical/Electrical Sensors/Voltage Sensor
  engine_rpm : Gain  Commented=on  Gain=4.5*(60/(2*pi))
  wheel_omega : Gain  Commented=on  Gain=1/(3.6*0.28)
  tag scope: ICE=global, Vdc=global, W=global, acc=global, assist_on=global, idc=global
  wires:
  Vdc Request/1 -> EM Controller/1(VdcRequest)
  DCDC Controller/1(G) -> DCDC Buck Converter/1(G)
  EM Controller/1(S) -> Gate Driver/1(S)
  [Vdc] -> EM Controller/7(Vdc_sens)
  Sensor ICE Shaft/2(A) -> Goto5/1
  Sensor ICE Shaft/1(W) -> ICE/1(w), [W]
  [W] -> EM Controller/5(w_sens)
  From2/1 -> EM Controller/6(th_sens)
  [iabc] -> EM Controller/4(iabc_sens)
  DCDC Buck Converter/1(vdc) -> DCDC Controller/2(Vdc)
  Constant/1 -> DCDC Controller/1(Ref)
  ICE/1(On) -> [ICE]
  [ICE] -> EM Controller/3(On)
  Step 12V Load/1 -> Switch 12V Load/1(S)
  PS-Simulink Converter5/1 -> [Vdc]
  Sensor ICE Shaft/3(acc) -> [acc]
  Transport Delay/1 -> ICE/2(Ref)
  ICE/2(Assist) -> [assist_on]
  [assist_on] -> EM Controller/2(Assist)
  PS-Simulink Converter1/1 -> [idc]
  Reference Speed/1 -> MATLAB Function/1(V_kmph), Gain1/1
  Product/1 -> Gain/1
  MATLAB Function/1(gear_ratio) -> Product/1
  Gain1/1 -> Product/2
  IDC drive-cycle/1 -> wheel_omega/1
  wheel_omega/1 -> engine_rpm/1
  engine_rpm/1 -> Saturation/1
  IDC reference/1 -> Transport Delay/1
  [soc] -> ICE/3(Soc_batt)
  Mux3/1 -> EM Controller/8(T_measured)
  [TC] -> Mux3/3  "C winding"
  [TB] -> Mux3/2  "B winding"
  [TA] -> Mux3/1  "A winding"
  [TR] -> Mux3/4  "Rotor"
  [Tbatt] -> Mux3/5  "Battery"
  Step 12V/1 -> Switch Load/1(S)
  From6/1 -> Low-Batt_cutoff/1(S)
  connections:
  Sensor ICE Torque/RConn1 -- ICE/RConn1 -- Sensor ICE Shaft/LConn1
  MRRef/LConn1 -- ISG/RConn2
  Converter/LConn1 -- Gate Driver/RConn1
  R1/RConn1 -- ERef DC/LConn1 -- R2/RConn1 -- Battery1/RConn1 -- DCDC Buck Converter/RConn2
  Sensor ICE Torque/LConn1 -- ISG/RConn1
  Converter/LConn2 -- Sensor Phase Currents/LConn1
  ISG/LConn1 -- Sensor Phase Currents/RConn1
  Switch Load/RConn1 -- RL/LConn1
  Switch 12V Load/RConn1 -- R2/LConn1
  R1/LConn1 -- Battery1/LConn1 -- Switch 12V Load/LConn1 -- DCDC Buck Converter/RConn1
  C2/RConn1 -- Electrical Reference/LConn1 -- Voltage Sensor/RConn2 -- Battery (System-Level)/RConn1 -- RL/RConn1 -- Solver Configuration/RConn1 -- Converter/RConn2 -- C1/RConn1 -- DCDC Buck Converter/LConn2
  C2/LConn1 -- Current Sensor/LConn1 -- Voltage Sensor/LConn1 -- Switch Load/LConn1 -- Converter/RConn1 -- C1/LConn1 -- DCDC Buck Converter/LConn1
  PS-Simulink Converter5/LConn1 -- Voltage Sensor/RConn1
  Thermal model/RConn1 -- ISG/RConn5
  Thermal model/RConn2 -- ISG/RConn4
  Thermal model/RConn3 -- ISG/RConn3
  Thermal model/LConn1 -- ISG/LConn2
  ThRef/LConn1 -- Temperature Source/RConn2
  Temperature Source/LConn1 -- Convective Heat Transfer/RConn1 -- Thermal model/LConn2
  Ambient Temperature/RConn1 -- Temperature Source/RConn1
  Current Sensor/RConn1 -- PS-Simulink Converter1/LConn1
  Convective Heat Transfer/LConn1 -- Battery (System-Level)/RConn2 -- Sensing Temperature/LConn1
  Battery (System-Level)/LConn1 -- Current Sensor/RConn2
